simulink model "DAQTest2"  (Simulink 7.9)
settings: Solver=FixedStepDiscrete  StartTime=0.0  StopTime=inf  FixedStep=0.001  RelTol=1e-3
undefined symbols (not defined in the file or in its folder): CalibrationParams, EncoderAngleLimits, EncoderThreshold, IMUAngleLimits, IMUThreshold, MotorParams
libraries: xpcethercatlib x160, marlo_lib_v01 x3, simulink x3, dspswit3 x1, xpclib x1
(part 3 of 3)

== matlab function DAQ_WITH_SAFETY/SAFETY ==
  data: MotorCurrentCommand input double; MotorCurrentCommandSafe output double; MedullaCommand input double; IMUCommand input double; q input double; dq input double; Switches input double; Thermistors input double; MedullaCommandSafe output double; IMUCommandSafe output double; SafetyStateOut output double; LogicVoltage input double; SafetyCountIn input double; SafetyCountOut output double
function [MotorCurrentCommandSafe, MedullaCommandSafe, IMUCommandSafe, SafetyStateOut, SafetyCountOut] = SafetyCheck(MotorCurrentCommand, MedullaCommand, IMUCommand, q, dq, Switches, Thermistors, LogicVoltage, SafetyCountIn)
    %#codegen
    
    % Checks DAQ inputs and outputs to ensure that the commands sent to the
    % robot and the state reported by the robot are okay. Any invalid
    % commands to the robot are discarded, and default (zero) commands are
    % send instead. The cause of the failure can be traced by logging the
    % SafetyStateOut output.
    %
    % SafetyStateOut is a double so that it can be logged efficiently in
    % the same array as the other outputs. However, we set individual bits
    % of the significand to encode various error states. Since the uint64
    % data type is not supported for code generation, we are limited to
    % using 32 bits of the significand. Thus the safety state should be an
    % integer in the range 0 to 2^32-1.
    
    % SAFE OUTPUTS
    % THESE OUTPUTS ARE USED IN A HARD SHUTDOWN, AND CAUSE ALL COMMANDED
    % CURRENTS TO BE ZEROED AND THE MEDULLAS TO ENTER THE ERROR STATE.
    MotorCurrentCommandSafe   = [0; 0; 0; 0; 0; 0];
    MedullaCommandSafe        = 5; % 5=ERROR (eStop)
    IMUCommandSafe            = 0;
    SafetyState               = uint32(0);
    
    % HARD SAFETY PARAMETERS
    % THE FOLLOWING PARAMETERS SPECIFY LIMITS WHICH, WHEN EXCEEDED, CAUSE
    % THE SAFETY TO LOCK DOWN THE ROBOT BY SENDING THE DEFAULT SAFE OUTPUTS
    % ABOVE.
    MAX_MOTOR_TEMP         = 80; % C
    MAX_MOTOR_CURRENT      = 120;  % Amps 
    VALID_MEDULLA_COMMANDS = [0 1 2 3 4 5 6 7];
    %VALID_IMU_COMMANDS     = [0 1 2]; % Meaningless for now
    
    MAX_TORSO_PITCH         = 30; % degrees
    MAX_TORSO_ROLL          = 30; % degrees
    MAX_LEG_ANGLE_DEVIATION = 50; % degrees from 180
    MAX_KNEE_ANGLE          = 100; % degrees; mechanical limit is 160 degrees
    MIN_KNEE_ANGLE          = 14.5; %22.5; % degrees; mechanical limit is reported to be 34.5 degrees
    MAX_LEG_LINK_FLEXION    = 85; % degrees from 180; mechanical limit is 107.5 degrees
    MAX_LEG_LINK_EXTENSION  = 30; % degrees from 180; mechanical limit is 45 degrees 
    % END (HARD SAFETY PARAMETERS)
    
    % SOFT SAFETY PARAMETERS
    % THE FOLLOWING PARAMETERS SPECIFY LIMITS WHICH DO NOT CAUSE THE SAFETY
    % TO LOCK DOWN THE WHOLE ROBOT. INSTEAD, APPROPRIATE CURENTS ARE
    % LIMITED TO PREVENT DRIVING THE MOTORS IN A MANNER THAT MIGHT CAUSE
    % DAMAGE
    MAX_HIP_ANGLE_SOFT           = 7; % degrees; mechanical limit is reported to be 20 degrees
    MIN_HIP_ANGLE_SOFT           = -15; % degrees; mechanical limit is reported to be -10 degrees 
    
    SOFT_LIMIT_WIDTH_HIP         = 4;  % degrees
    SOFT_LIMIT_UMAX_HIP          = 15; % Amps
    % END (SOFT SAFETY PARAMETERS)
    
    
    % SAFETY STATE DEFINITION
    SSMASK_INVALID_MOTOR_COMMAND   = uint32(1);
    SSMASK_INVALID_MEDULLA_COMMAND = uint32(2);
    SSMASK_INVALID_IMU_COMMAND     = uint32(4);
    SSMASK_BAD_CONFIGURATION       = uint32(8);
    SSMASK_OVERTEMP                = uint32(256);   % Each motor will set one bit of second byte
    SSMASK_LIMSWITCH               = uint32(65536); 
    
    %{
    % CHECK THERMISTORS    
    SafetyState = bitor(SafetyState, bitshift(SSMASK_OVERTEMP, 0)*uint32(any(Thermistors(1:6)  >MAX_MOTOR_TEMP)));
    SafetyState = bitor(SafetyState, bitshift(SSMASK_OVERTEMP, 1)*uint32(any(Thermistors(7:12) >MAX_MOTOR_TEMP)));
    SafetyState = bitor(SafetyState, bitshift(SSMASK_OVERTEMP, 2)*uint32(any(Thermistors(13:15)>MAX_MOTOR_TEMP)));
    SafetyState = bitor(SafetyState, bitshift(SSMASK_OVERTEMP, 3)*uint32(any(Thermistors(16:21)>MAX_MOTOR_TEMP)));
    SafetyState = bitor(SafetyState, bitshift(SSMASK_OVERTEMP, 4)*uint32(any(Thermistors(22:27)>MAX_MOTOR_TEMP)));
    SafetyState = bitor(SafetyState, bitshift(SSMASK_OVERTEMP, 5)*uint32(any(Thermistors(28:30)>MAX_MOTOR_TEMP)));
    %}
    
    %{
    % CHECK LIMIT SWITCHES
    SafetyState = bitor(SafetyState, bitshift(SSMASK_LIMSWITCH, 0)*uint32(any(Thermistors(1:6)  >MAX_MOTOR_TEMP)));
    SafetyState = bitor(SafetyState, bitshift(SSMASK_LIMSWITCH, 1)*uint32(any(Thermistors(7:12) >MAX_MOTOR_TEMP)));
    SafetyState = bitor(SafetyState, bitshift(SSMASK_LIMSWITCH, 2)*uint32(any(Thermistors(13:15)>MAX_MOTOR_TEMP)));
    SafetyState = bitor(SafetyState, bitshift(SSMASK_LIMSWITCH, 3)*uint32(any(Thermistors(16:21)>MAX_MOTOR_TEMP)));
    SafetyState = bitor(SafetyState, bitshift(SSMASK_LIMSWITCH, 4)*uint32(any(Thermistors(22:27)>MAX_MOTOR_TEMP)));
    SafetyState = bitor(SafetyState, bitshift(SSMASK_LIMSWITCH, 5)*uint32(any(Thermistors(28:30)>MAX_MOTOR_TEMP)));
    %}
    
    % VALIDATE MOTOR COMMAND
    if any(~isfinite(MotorCurrentCommand)) ...                    % Check for NaN and +Inf and -Inf
            || any(abs(MotorCurrentCommand) > MAX_MOTOR_CURRENT)  % Check for extremely large commands
        
        SafetyState = bitor(SafetyState, SSMASK_INVALID_MOTOR_COMMAND);
    end
    
    % VALIDATE MEDULLA COMMAND
    if any(~ismember(MedullaCommand, VALID_MEDULLA_COMMANDS))
        SafetyState = bitor(SafetyState, SSMASK_INVALID_MEDULLA_COMMAND);
    end
    
    % VALIDATE IMU COMMAND
    %if any(~ismember(IMUCommand, VALID_IMU_COMMANDS))
    %    SafetyState = bitor(SafetyState, SSMASK_INVALID_IMU_COMMAND);
    %end
    
    
    % CHECK ROBOT CONFIGURATION (HARD SAFETY)   

    % THE FOLLOWING LIMITS, WHEN EXCEEDED, CAUSE THE SAFETY TO LOCK DOWN
    % THE ROBOT BY SENDING THE DEFAULT SAFE OUTPUTS ABOVE.
    qyT = q(2);
    qxT = q(3);
    qLA = [0 0 0 0.5 0.5   0   0 0 0 0 0 0 0; ...
           0 0 0   0   0 0.5 0.5 0 0 0 0 0 0]*q;
	qKA = [0 0 0  -1   1   0   0 0 0 0 0 0 0; ...
           0 0 0   0   0  -1   1 0 0 0 0 0 0]*q;
    qLegLinkFlexion = [0 0 0  -1   0   0   0 0 0 0 0 0 0; ...
                       0 0 0   0   1   0   0 0 0 0 0 0 0; ...
                       0 0 0   0   0  -1   0 0 0 0 0 0 0
                       0 0 0   0   0   0   1 0 0 0 0 0 0]*q + [1; -1; 1; -1]*pi;
                   
    if abs(qxT) > MAX_TORSO_PITCH*pi/180 ...
            || abs(qyT) > MAX_TORSO_ROLL*pi/180 ...
            || any(abs(qLA-pi) > MAX_LEG_ANGLE_DEVIATION*pi/180) ...
            || any(qKA > MAX_KNEE_ANGLE*pi/180) ...
            || any(qKA < MIN_KNEE_ANGLE*pi/180) ...
            || any(qLegLinkFlexion > MAX_LEG_LINK_FLEXION*pi/180) ...
            || any(qLegLinkFlexion < -MAX_LEG_LINK_EXTENSION*pi/180)
        
        SafetyState = bitor(SafetyState, SSMASK_BAD_CONFIGURATION);
    end
        
    
    % CHECK ROBOT CONFIGURATION (SOFT SAFETY)
    
    % THE FOLLOWING LIMITS, WHEN EXCEEDED, DO *NOT* CAUSE THE SAFETY TO
    % LOCK DOWN THE WHOLE ROBOT. INSTEAD, APPROPRIATE CURENTS ARE LIMITED
    % TO PREVENT DRIVING THE MOTORS IN A MANNER THAT MIGHT CAUSE DAMAGE
    q3R = q(10);
    q3L = q(13);
    
    MotorCurrentCommand(3) = continuouslySaturate(MotorCurrentCommand(3), q3R, [MIN_HIP_ANGLE_SOFT MAX_HIP_ANGLE_SOFT]*pi/180, SOFT_LIMIT_WIDTH_HIP*pi/180, SOFT_LIMIT_UMAX_HIP);
    MotorCurrentCommand(6) = continuouslySaturate(MotorCurrentCommand(6), q3L, [MIN_HIP_ANGLE_SOFT MAX_HIP_ANGLE_SOFT]*pi/180, SOFT_LIMIT_WIDTH_HIP*pi/180, SOFT_LIMIT_UMAX_HIP);
    
    
    % The SafetyState output must be a double for efficient storage in an array with other DAQ outputs
    SafetyStateOut = double(SafetyState); 
    
    % IF EVERYTHING LOOKS OKAY (SAFETYSTATE==0), THEN PASS THE COMMANDS TO THE DAQ
    if (SafetyState==0)
        SafetyCountOut = max(0, SafetyCountIn-1);
    else
        SafetyCountOut = min(SafetyCountIn+1, 10);
    end
    
    if (SafetyStateOut<10)
        MotorCurrentCommandSafe = MotorCurrentCommand;
        MedullaCommandSafe = MedullaCommand;
        IMUCommandSafe = IMUCommand;
    end
end
